simulink model "RoadProfile"  (R2019a)
settings: Solver=VariableStepAuto  StartTime=0.0  StopTime=60  RelTol=1e-3
libraries: simulink_extras x2
settings Model: Creator=Owen Heaney  LastModifiedBy=Owen Heaney

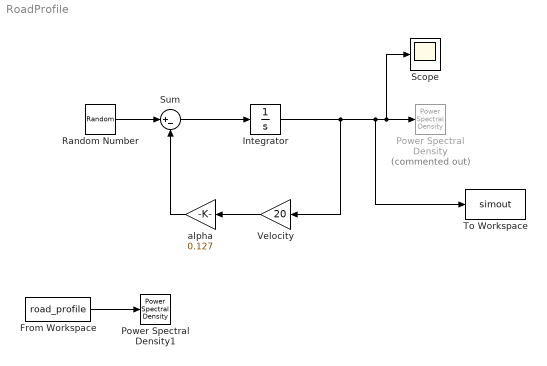
== system RoadProfile ==
  From Workspace : FromWorkspace  VariableName=road_profile  SampleTime=0
  Integrator : Integrator
  Power Spectral Density : simulink_extras/Additional Sinks/Power Spectral Density  Commented=on  npts=1280  fftpts=51200  HowOften=64  sampleT=0.1
      settings: SourceProductName=Simulink  SourceProductBaseCode=SL
  Power Spectral Density1 : simulink_extras/Additional Sinks/Power Spectral Density  npts=500  fftpts=20000  HowOften=64  sampleT=0.1
      settings: SourceProductName=Simulink  SourceProductBaseCode=SL
  Random Number : RandomNumber  Variance=0.002  SampleTime=0.1
  Scope : Scope
  Sum : Sum  Inputs=|+-
  To Workspace : ToWorkspace  VariableName=simout  SaveFormat=Timeseries  SampleTime=-1
  Velocity : Gain  Gain=20
  alpha : Gain  Gain=0.127
  wires:
  Random Number/1 -> Sum/1
  Sum/1 -> Integrator/1
  Integrator/1 -> To Workspace/1, Scope/1, Power Spectral Density/1, Velocity/1
  Velocity/1 -> alpha/1
  alpha/1 -> Sum/2
  From Workspace/1 -> Power Spectral Density1/1
